simulink model "PIL"  (R2023a)
settings: Solver=VariableStepAuto  StartTime=0.0  StopTime=1  RelTol=1e-3
values from neighbouring files (symbols this model uses):
  des_pos = deg2rad(45)    [controller_design.m]
  V_0 = 0.2    [controller_design.m]
libraries: cstblocks x2
settings Model: Creator=m250246  LastModifiedBy=m250246

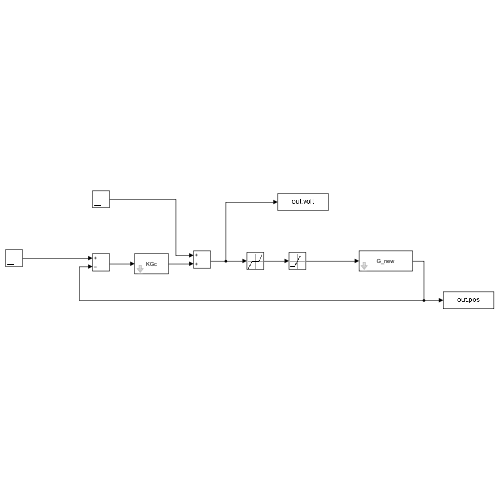
[thumbnail: Simulink's stored preview of the top-level diagram]
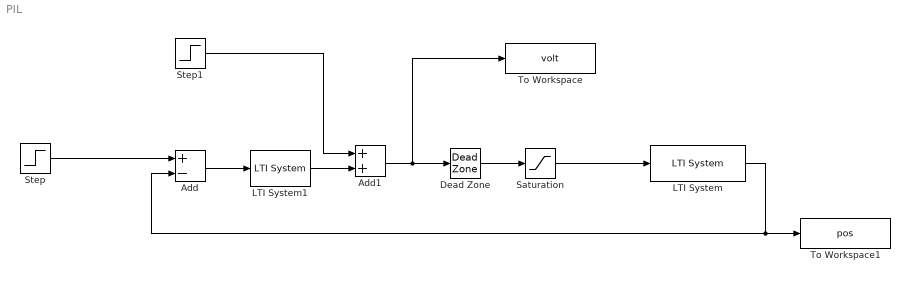
== system PIL ==
  Add : Sum  Inputs=+-
  Add1 : Sum
  Dead Zone : DeadZone  LowerValue=-V_0  UpperValue=V_0
  LTI System : cstblocks/LTI System  sys=G_new  IC=[]
  LTI System1 : cstblocks/LTI System  sys=KGc  IC=[]
  Saturation : Saturate  UpperLimit=1 - V_0  LowerLimit=-(1-V_0)
  Step : Step  Time=0  After=des_pos  SampleTime=0
  Step1 : Step  Time=0  After=V_0  SampleTime=0
  To Workspace : ToWorkspace  VariableName=volt  SaveFormat=Timeseries  SampleTime=-1
  To Workspace1 : ToWorkspace  VariableName=pos  SaveFormat=Timeseries  SampleTime=-1
  wires:
  LTI System/1 -> Add/2, To Workspace1/1
  LTI System1/1 -> Add1/2
  Add/1 -> LTI System1/1
  Step/1 -> Add/1
  Saturation/1 -> LTI System/1
  Step1/1 -> Add1/1
  Dead Zone/1 -> Saturation/1
  Add1/1 -> To Workspace/1, Dead Zone/1
